simulink model "rc_blink_sim"  (R2017a)
settings: Solver=FixedStepAuto  StartTime=0.0  StopTime=30.0  RelTol=1e-3  EnableMultiTasking=on
libraries: simulink x6
settings Model: SimulationMode=external  Creator=Parker  LastModifiedBy=Parker
settings SolverCC: PositivePriorityOrder=on
settings OptimizationCC: PassReuseOutputArgsAs=Individual arguments  MaxStackSize=64
settings DebuggingCC: ParameterTunabilityLossMsg=error
settings HardwareCC: ProdBitPerPointer=32  ProdBitPerSizeT=32  ProdBitPerPtrDiffT=32  ProdLargestAtomicInteger=Long  ProdLargestAtomicFloat=Double  ProdWordSize=32  ProdHWDeviceType=ARM Compatible->ARM Cortex
settings SFSimCC: MATLABDynamicMemAlloc=off
settings RTWCC: SystemTargetFile=ert.tlc  HardwareBoard=Raspberry Pi  TLCOptions="-aInlineSetEventsForThisBaseRateFcn=TLC_FALSE -aSuppressMultiTaskScheduler=TLC_FALSE  -aRateBasedStepFcn=0"  TemplateMakefile=ert_default_tmf  Description=Embedded Coder  GenerateReport=on  Toolchain=GNU GCC Raspberry Pi  IncludeHyperlinkInReport=on  LaunchReport=on  GenerateTraceInfo=on  GenerateTraceReport=on  GenerateTraceReportSl=on  GenerateTraceReportSf=on  GenerateTraceReportEml=on
settings CodeAppCC: ForceParamTrailComments=on  IgnoreCustomStorageClasses=off  OperatorAnnotations=on  SimulinkDataObjDesc=on  SFDataObjDesc=on  MATLABFcnDesc=on  InsertBlockDesc=on  MATLABSourceComments=on
settings ERTTargetCC: SupportVariableSizeSignals=on

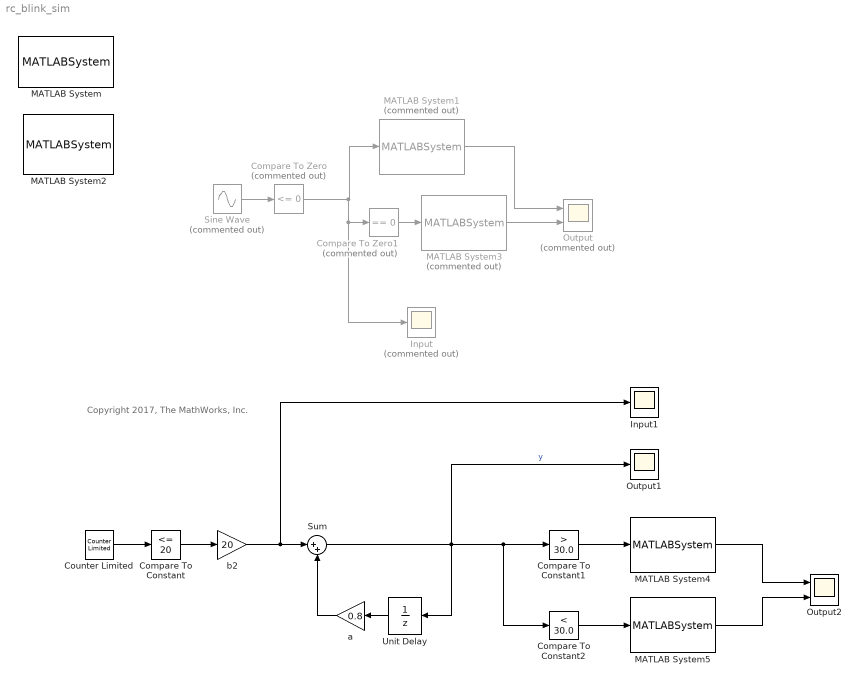
== system rc_blink_sim ==
  note: Copyright 2017, The MathWorks, Inc.
  Compare To Constant : simulink/Logic and Bit Operations/Compare To Constant  relop=<=  const=20  OutDataTypeStr=uint8
  Compare To Constant1 : simulink/Logic and Bit Operations/Compare To Constant  relop=>  const=30.0  OutDataTypeStr=uint8
  Compare To Constant2 : simulink/Logic and Bit Operations/Compare To Constant  relop=<  const=30.0  OutDataTypeStr=uint8
  Compare To Zero : simulink/Logic and Bit Operations/Compare To Zero  Commented=on  relop=<=  OutDataTypeStr=uint8
  Compare To Zero1 : simulink/Logic and Bit Operations/Compare To Zero  Commented=on  relop===  OutDataTypeStr=uint8
  Counter Limited : simulink/Sources/Counter Limited  uplimit=40  tsamp=0.1
  Input : Scope  Commented=on
  Input1 : Scope
  MATLAB System : MATLABSystem  System=rc_initialize_sys
      mask Type: rc_initialize_sys
      mask Display: disp('rc_initialize_sys');
  MATLAB System1 : MATLABSystem  Commented=on  System=rc_set_led  rc_led_t=1
      mask Type: rc_set_led
      mask Display:
      | disp('rc_set_led');
      | port_label('input',1,'u');
      | port_label('output',1,'y');
  MATLAB System2 : MATLABSystem  System=rc_cleanup_sys
      mask Type: rc_cleanup_sys
      mask Display: disp('rc_cleanup_sys');
  MATLAB System3 : MATLABSystem  Commented=on  System=rc_set_led  rc_led_t=0
      mask Type: rc_set_led
      mask Display:
      | disp('rc_set_led');
      | port_label('input',1,'u');
      | port_label('output',1,'y');
  MATLAB System4 : MATLABSystem  System=rc_set_led  rc_led_t=0
      mask Type: rc_set_led
      mask Display:
      | disp('rc_set_led');
      | port_label('input',1,'u');
      | port_label('output',1,'y');
  MATLAB System5 : MATLABSystem  System=rc_set_led  rc_led_t=1
      mask Type: rc_set_led
      mask Display:
      | disp('rc_set_led');
      | port_label('input',1,'u');
      | port_label('output',1,'y');
  Output : Scope  Commented=on  NumInputPorts=2
  Output1 : Scope
  Output2 : Scope  NumInputPorts=2
  Sine Wave : Sin  Commented=on  SineType=Sample based  Amplitude=20  Frequency=2  Samples=20  SampleTime=0.1
  Sum : Sum  Inputs=|++
  Unit Delay : UnitDelay  SampleTime=-1
  a : Gain  Gain=0.8  SaturateOnIntegerOverflow=on  OutDataTypeStr=Inherit: Same as input  ParamDataTypeStr=Inherit: Same as input
  b2 : Gain  Gain=20  ParamDataTypeStr=double  OutDataTypeStr=double  SaturateOnIntegerOverflow=on
  wires:
  Sine Wave/1 -> Compare To Zero/1
  Compare To Zero/1 -> Compare To Zero1/1, Input/1, MATLAB System1/1
  MATLAB System1/1 -> Output/1
  MATLAB System3/1 -> Output/2
  Compare To Zero1/1 -> MATLAB System3/1
  Counter Limited/1 -> Compare To Constant/1
  b2/1 -> Input1/1, Sum/1
  a/1 -> Sum/2
  Sum/1 -> Unit Delay/1, Output1/1, Compare To Constant2/1, Compare To Constant1/1  "y"
  Unit Delay/1 -> a/1
  Compare To Constant/1 -> b2/1
  Compare To Constant1/1 -> MATLAB System4/1
  Compare To Constant2/1 -> MATLAB System5/1
  MATLAB System4/1 -> Output2/1
  MATLAB System5/1 -> Output2/2
